simulink model "AWE_Model"  (R2020a)
settings: Solver=VariableStepAuto  StartTime=0.0  StopTime=10.0  RelTol=1e-3
values from neighbouring files (symbols this model uses):
  G_vWind = [10;0;0]    [AWE_Model_ts.m]
  thrDL = 0    [AWE_Model_ts.m]
  thrL = norm(init_G_rKite)    [AWE_Model_ts.m]
libraries: flightController_cl x1, plantModel_cl x1
settings Model: Creator=Ayaz  LastModifiedBy=Ayaz

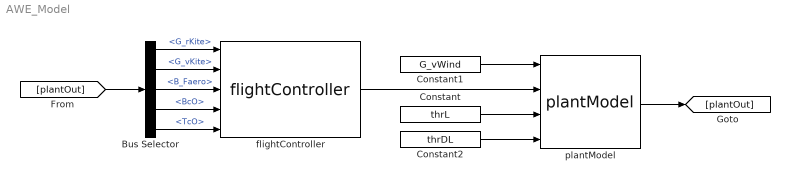
== system AWE_Model ==
  Bus Selector : BusSelector  OutputSignals=G_rKite,G_vKite,B_Faero,BcO,TcO
  Constant : Constant  Value=thrL
  Constant1 : Constant  Value=G_vWind
  Constant2 : Constant  Value=thrDL
  flightController : flightController_cl/flightController  PW=60  PH=28  PE=30  L1=0.05  initialPathParam=0  kiteMass=36.8  kp=1  ki=0  kd=0  tau=0.1
  plantModel : plantModel_cl/plantModel  kiteMass=36.8  kiteJmat=eye(3)  refChord=0.55  refSpan=5.5  refArea=3  xme_0=[0 0 0]  Vm_0=[0 0 0]  eul_0=[0 0 0]  pm_0=[0 0 0]  dThr=0  CdThr=0  thrSpringCns=10243  rhoAir=1.225  gravAccl=0
  wires:
  plantModel/1 -> [plantOut]
  [plantOut] -> Bus Selector/1
  Bus Selector/1 -> flightController/1  "<G_rKite>"
  Bus Selector/2 -> flightController/2  "<G_vKite>"
  Bus Selector/3 -> flightController/3  "<B_Faero>"
  Bus Selector/4 -> flightController/4  "<BcO>"
  Bus Selector/5 -> flightController/5  "<TcO>"
  flightController/1 -> plantModel/2
  Constant/1 -> plantModel/3
  Constant1/1 -> plantModel/1
  Constant2/1 -> plantModel/4
